simulink model "gantry_crane_model"  (R2024a)
settings: Solver=VariableStepAuto  StartTime=0.0  StopTime=150  RelTol=1e-3
values from neighbouring files (symbols this model uses):
  constant_tq_time = 80    [gantry_crane.m]
  endTime = constant_tq_time + 2*startTime    (= 120)    [gantry_crane.m]
  finalTime = constant_tq_time + startTime    (= 100)    [gantry_crane.m]
  g = 9.81    [gantry_crane.m]
  l = 8    [gantry_crane.m]
  max_torque = 200    [gantry_crane.m]
  mC = 8 * 1000    (= 8000)    [gantry_crane.m]
  mL = 25 * 1000    (= 25000)    [gantry_crane.m]
  slop = 10    [gantry_crane.m]
  startTime = max_torque/slop    (= 20)    [gantry_crane.m]
libraries: simulink x2
settings Model: Creator=harsh  LastModifiedBy=harsh
settings RTWCC: GPUComputeCapability=3.5

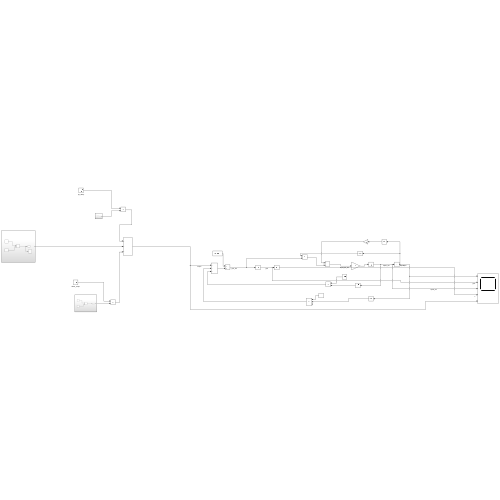
[thumbnail: Simulink's stored preview of the top-level diagram]
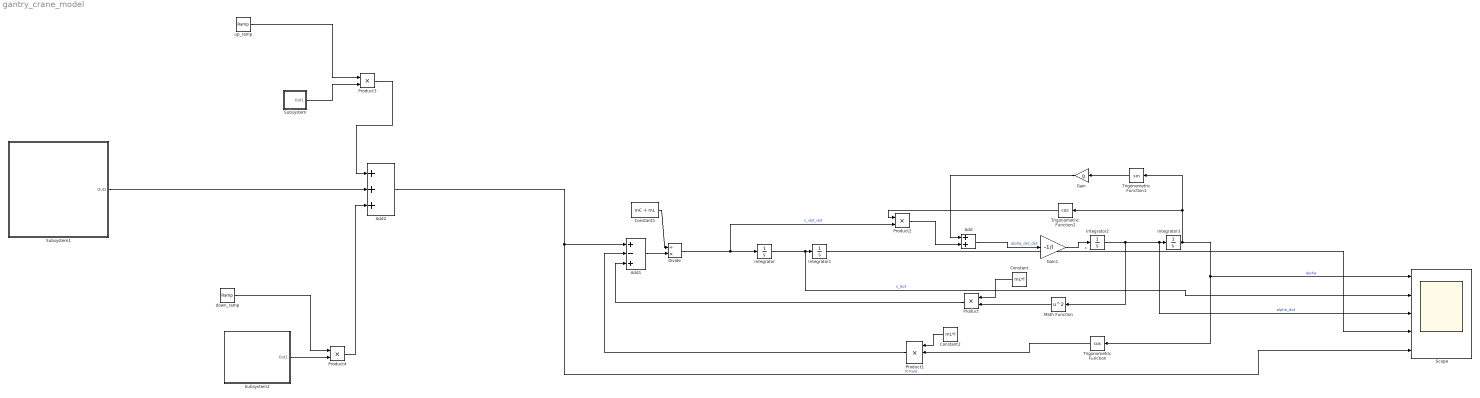
== system gantry_crane_model ==
  Add : Sum
  Add1 : Sum  Inputs=+-+
  Add2 : Sum  Inputs=+++
  Constant : Constant  Value=mL*l
  Constant1 : Constant  Value=mC + mL
  Constant2 : Constant  Value=mL*l
  Divide : Product  Inputs=/*
  Gain : Gain  Gain=g
  Gain1 : Gain  Gain=-1/l
  Integrator{,1..3} (4 alike) : Integrator
  Math Function : Math  Operator=square
  Product{,2..4} (4 alike) : Product
  Product1 : Product  Inputs=3
  Scope : Scope  NumInputPorts=5
  Subsystem : Subsystem
  Subsystem1 : Subsystem
  Subsystem2 : Subsystem
  Trigonometric Function : Trigonometry  Operator=cos
  Trigonometric Function1 : Trigonometry
  Trigonometric Function2 : Trigonometry  Operator=cos
  down_ramp : simulink/Sources/Ramp  slope=-slop  start=startTime+constant_tq_time  InitialOutput=max_torque
  up_ramp : simulink/Sources/Ramp  slope=slop  start=0  InitialOutput=0
  wires:
  Divide/1 -> Product2/2, Integrator/1  "x_dot_dot"
  Integrator/1 -> Scope/2, Integrator1/1  "x_dot"
  Integrator1/1 -> Scope/4  "x"
  Add/1 -> Gain1/1  "alpha_dot_dot"
  Integrator2/1 -> Math Function/1, Scope/3, Integrator3/1  "alpha_dot"
  Integrator3/1 -> Trigonometric Function1/1, Trigonometric Function2/1, Trigonometric Function/1, Scope/1  "alpha"
  Constant/1 -> Product/1
  Math Function/1 -> Product/2
  Constant2/1 -> Product1/1
  Trigonometric Function/1 -> Product1/2
  Product/1 -> Add1/3
  Constant1/1 -> Divide/1
  Add1/1 -> Divide/2
  Product1/1 -> Add1/2
  Add2/1 -> Scope/5, Add1/1  "torque"
  Trigonometric Function1/1 -> Gain/1
  Trigonometric Function2/1 -> Product2/1
  Gain/1 -> Add/1
  Product2/1 -> Add/2
  Gain1/1 -> Integrator2/1
  Subsystem1/1(Out1) -> Add2/2
  up_ramp/1 -> Product3/1
  Subsystem/1(Out1) -> Product3/2
  Subsystem2/1(Out1) -> Product4/2
  down_ramp/1 -> Product4/1
  Product3/1 -> Add2/1
  Product4/1 -> Add2/3

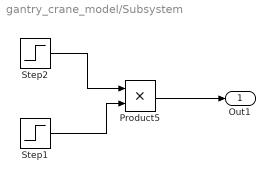
== system gantry_crane_model/Subsystem ==
  Product5 : Product
  Step1 : Step  Time=startTime  Before=1  After=0  SampleTime=0
  Step2 : Step  Time=0  SampleTime=0
  Out1 : Outport
  wires:
  Step2/1 -> Product5/1
  Step1/1 -> Product5/2
  Product5/1 -> Out1/1

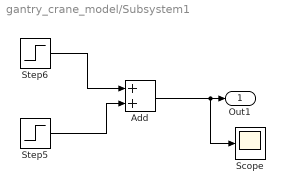
== system gantry_crane_model/Subsystem1 ==
  Add : Sum
  Scope : Scope
  Step5 : Step  Time=finalTime  After=-max_torque  SampleTime=0
  Step6 : Step  Time=startTime  After=max_torque  SampleTime=0
  Out1 : Outport
  wires:
  Add/1 -> Scope/1, Out1/1
  Step5/1 -> Add/2
  Step6/1 -> Add/1

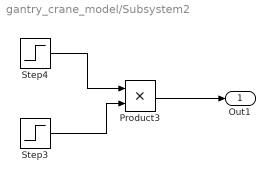
== system gantry_crane_model/Subsystem2 ==
  Product3 : Product
  Step3 : Step  Time=endTime  Before=1  After=0  SampleTime=0
  Step4 : Step  Time=finalTime  SampleTime=0
  Out1 : Outport
  wires:
  Step3/1 -> Product3/2
  Step4/1 -> Product3/1
  Product3/1 -> Out1/1
